simulink model "db_pino_crem"  (R2018a)
settings: Solver=VariableStepAuto  StartTime=0.0  StopTime=1.6  RelTol=1e-3
values from neighbouring files (symbols this model uses):
  A = [0 1 ... (first row only)    [ejemplo_engranajes.m]
  B = [0 0 ... (first row only)    [ejemplo_engranajes.m]
  B1 = 450    [ejemplo_engranajes.m]
  B2 = 200    [ejemplo_engranajes.m]
  C = [1 0]    [ejemplo_engranajes.m]
  D = zeros(1,2)    [ejemplo_engranajes.m]
undefined symbols (not defined in the file or in its folder): J, K, M, R
settings Model: Creator=carma  LastModifiedBy=carma

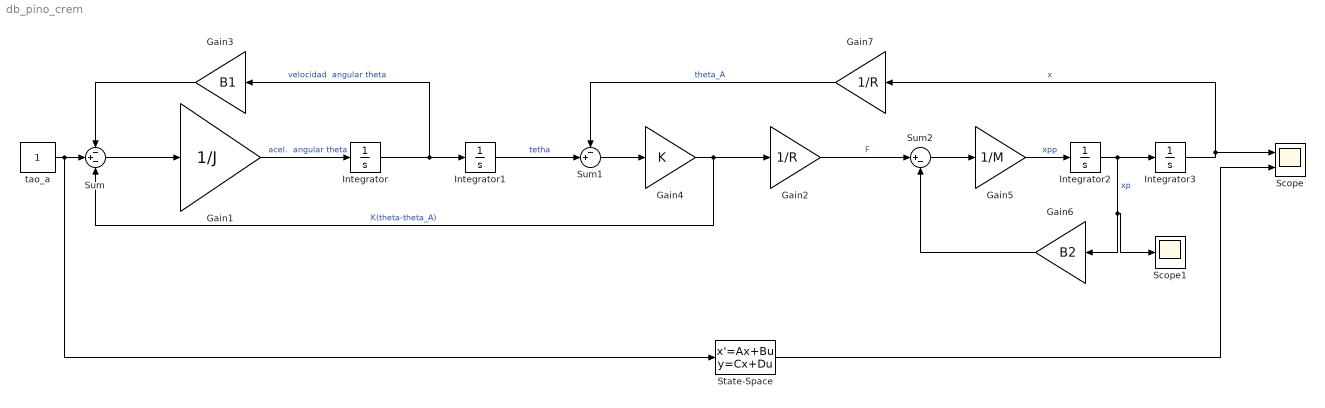
== system db_pino_crem ==
  Gain1 : Gain  Gain=1/J
  Gain2 : Gain  Gain=1/R
  Gain3 : Gain  Gain=B1
  Gain4 : Gain  Gain=K
  Gain5 : Gain  Gain=1/M
  Gain6 : Gain  Gain=B2
  Gain7 : Gain  Gain=1/R
  Integrator{,1..3} (4 alike) : Integrator
  Scope : Scope  NumInputPorts=2
  Scope1 : Scope
  State-Space : StateSpace  A=A  B=B  C=C  D=D  InitialCondition=0
  Sum : Sum  Inputs=-+-
  Sum1 : Sum  Inputs=-+|
  Sum2 : Sum  Inputs=|+-
  tao_a : Constant
  wires:
  Integrator2/1 -> Scope1/1, Gain6/1, Integrator3/1  "xp"
  Sum2/1 -> Gain5/1
  Gain4/1 -> Sum/3, Gain2/1  "K(theta-theta_A)"
  Sum/1 -> Gain1/1
  Gain1/1 -> Integrator/1  "acel.  angular theta"
  Integrator3/1 -> Gain7/1, Scope/1  "x"
  Gain5/1 -> Integrator2/1  "xpp"
  Integrator1/1 -> Sum1/2  "tetha"
  tao_a/1 -> State-Space/1, Sum/2
  Gain2/1 -> Sum2/1  "F"
  Gain6/1 -> Sum2/2
  Integrator/1 -> Gain3/1, Integrator1/1  "velocidad  angular theta"
  Sum1/1 -> Gain4/1
  Gain7/1 -> Sum1/1  "theta_A"
  Gain3/1 -> Sum/1
  State-Space/1 -> Scope/2
